simulink model "drone_pitch_test"  (R2025b)
settings: Solver=VariableStepAuto  StartTime=0.0  StopTime=3  RelTol=1e-3
libraries: sim3dcameralib x4, uavsim3dlib x4, sim3dautolib x1, sim3dlib x1
settings Model: Creator=lab  LastModifiedBy=lab

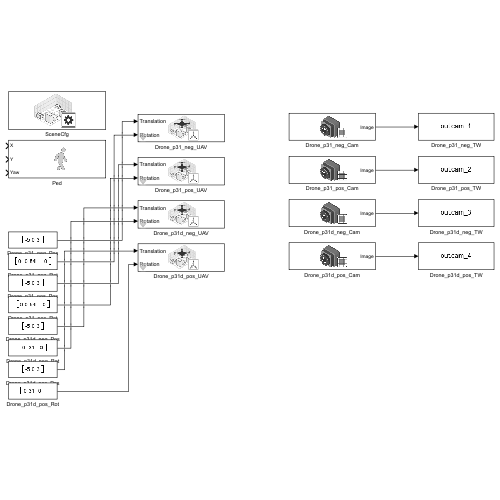
[thumbnail: Simulink's stored preview of the top-level diagram]
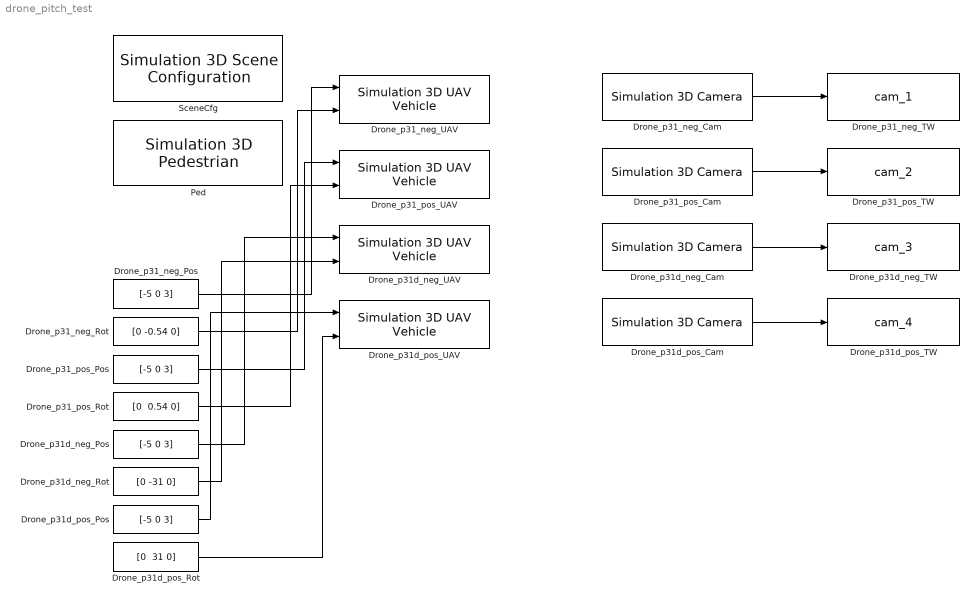
== system drone_pitch_test ==
  Drone_p31_neg_Cam : sim3dcameralib/Simulation 3D Camera  Priority=1  sensorTag=Sim3dSensor  sensorId=1  sensorName=Sim3dSensor  vehTagList={'Scene Origin', 'Drone_p31_neg'}  vehTag=Drone_p31_neg  CoordinateSystem=ISO8855  mountLoc=Origin  offsetFlag=on  tmountOffset=[0 0 0]  extTmount=off  rmountOffset=[0 0 0]  extRmount=off  FocalLength=[1109, 1109]  OpticalCenter=[640, 360]  ImageSize=[640 360]  RadialDistortion=[0, 0]  TangentialDistortion=[0, 0]  SensorSkew=0  VisualizeFieldOfView=off  FieldOfViewRange=61  DepthOutportEnabled=off  SemanticOutportEnabled=off  TransformOutportEnabled=off  SampleTime=0.5  mountPoint=[0 0 0]  mountOrientation=[0 0 0]  aMode=4  ID=1
      settings: LibrarySourceBlock=uavsim3dlib/Simulation 3D Camera
  Drone_p31_neg_Pos : Constant  Value=[-5 0 3]
  Drone_p31_neg_Rot : Constant  Value=[0 -0.54 0]
  Drone_p31_neg_TW : ToWorkspace  VariableName=cam_1  SaveFormat=Structure With Time  SampleTime=-1
  Drone_p31_neg_UAV : uavsim3dlib/Simulation 3D UAV Vehicle  Priority=-1  Mesh=Quadrotor  MeshPath=/MathWorksUAVContent/UAVs/HexaRotorUAV/HexaRotor.HexaRotor  Color=Red  ActorName=Drone_p31_neg  UseGlobalFrame=off  InitialTranslation=[-5 0 3]  InitialRotation=[0 -0.54 0]  InitialTranslationGlobal=[0 0 0]  InitialGeoOrigin=[0 0 0]  InitialRotationGlobal=[0 0 0]  SampleTime=-1  ActorType=SimulinkVehicle  ID=C  aMode=4  ActorTag=Drone_p31_neg
  Drone_p31_pos_Cam : sim3dcameralib/Simulation 3D Camera  Priority=1  sensorTag=Sim3dSensor  sensorId=2  sensorName=Sim3dSensor  vehTagList={'Scene Origin', 'Drone_p31_pos'}  vehTag=Drone_p31_pos  CoordinateSystem=ISO8855  mountLoc=Origin  offsetFlag=on  tmountOffset=[0 0 0]  extTmount=off  rmountOffset=[0 0 0]  extRmount=off  FocalLength=[1109, 1109]  OpticalCenter=[640, 360]  ImageSize=[640 360]  RadialDistortion=[0, 0]  TangentialDistortion=[0, 0]  SensorSkew=0  VisualizeFieldOfView=off  FieldOfViewRange=61  DepthOutportEnabled=off  SemanticOutportEnabled=off  TransformOutportEnabled=off  SampleTime=0.5  mountPoint=[0 0 0]  mountOrientation=[0 0 0]  aMode=4  ID=2
      settings: LibrarySourceBlock=uavsim3dlib/Simulation 3D Camera
  Drone_p31_pos_Pos : Constant  Value=[-5 0 3]
  Drone_p31_pos_Rot : Constant  Value="[0  0.54 0]"
  Drone_p31_pos_TW : ToWorkspace  VariableName=cam_2  SaveFormat=Structure With Time  SampleTime=-1
  Drone_p31_pos_UAV : uavsim3dlib/Simulation 3D UAV Vehicle  Priority=-1  Mesh=Quadrotor  MeshPath=/MathWorksUAVContent/UAVs/HexaRotorUAV/HexaRotor.HexaRotor  Color=Red  ActorName=Drone_p31_pos  UseGlobalFrame=off  InitialTranslation=[-5 0 3]  InitialRotation="[0  0.54 0]"  InitialTranslationGlobal=[0 0 0]  InitialGeoOrigin=[0 0 0]  InitialRotationGlobal=[0 0 0]  SampleTime=-1  ActorType=SimulinkVehicle  ID=C  aMode=4  ActorTag=Drone_p31_pos
  Drone_p31d_neg_Cam : sim3dcameralib/Simulation 3D Camera  Priority=1  sensorTag=Sim3dSensor  sensorId=3  sensorName=Sim3dSensor  vehTagList={'Scene Origin', 'Drone_p31d_neg'}  vehTag=Drone_p31d_neg  CoordinateSystem=ISO8855  mountLoc=Origin  offsetFlag=on  tmountOffset=[0 0 0]  extTmount=off  rmountOffset=[0 0 0]  extRmount=off  FocalLength=[1109, 1109]  OpticalCenter=[640, 360]  ImageSize=[640 360]  RadialDistortion=[0, 0]  TangentialDistortion=[0, 0]  SensorSkew=0  VisualizeFieldOfView=off  FieldOfViewRange=61  DepthOutportEnabled=off  SemanticOutportEnabled=off  TransformOutportEnabled=off  SampleTime=0.5  mountPoint=[0 0 0]  mountOrientation=[0 0 0]  aMode=4  ID=3
      settings: LibrarySourceBlock=uavsim3dlib/Simulation 3D Camera
  Drone_p31d_neg_Pos : Constant  Value=[-5 0 3]
  Drone_p31d_neg_Rot : Constant  Value=[0 -31 0]
  Drone_p31d_neg_TW : ToWorkspace  VariableName=cam_3  SaveFormat=Structure With Time  SampleTime=-1
  Drone_p31d_neg_UAV : uavsim3dlib/Simulation 3D UAV Vehicle  Priority=-1  Mesh=Quadrotor  MeshPath=/MathWorksUAVContent/UAVs/HexaRotorUAV/HexaRotor.HexaRotor  Color=Red  ActorName=Drone_p31d_neg  UseGlobalFrame=off  InitialTranslation=[-5 0 3]  InitialRotation=[0 -31 0]  InitialTranslationGlobal=[0 0 0]  InitialGeoOrigin=[0 0 0]  InitialRotationGlobal=[0 0 0]  SampleTime=-1  ActorType=SimulinkVehicle  ID=C  aMode=4  ActorTag=Drone_p31d_neg
  Drone_p31d_pos_Cam : sim3dcameralib/Simulation 3D Camera  Priority=1  sensorTag=Sim3dSensor  sensorId=4  sensorName=Sim3dSensor  vehTagList={'Scene Origin', 'Drone_p31d_pos'}  vehTag=Drone_p31d_pos  CoordinateSystem=ISO8855  mountLoc=Origin  offsetFlag=on  tmountOffset=[0 0 0]  extTmount=off  rmountOffset=[0 0 0]  extRmount=off  FocalLength=[1109, 1109]  OpticalCenter=[640, 360]  ImageSize=[640 360]  RadialDistortion=[0, 0]  TangentialDistortion=[0, 0]  SensorSkew=0  VisualizeFieldOfView=off  FieldOfViewRange=61  DepthOutportEnabled=off  SemanticOutportEnabled=off  TransformOutportEnabled=off  SampleTime=0.5  mountPoint=[0 0 0]  mountOrientation=[0 0 0]  aMode=4  ID=4
      settings: LibrarySourceBlock=uavsim3dlib/Simulation 3D Camera
  Drone_p31d_pos_Pos : Constant  Value=[-5 0 3]
  Drone_p31d_pos_Rot : Constant  Value="[0  31 0]"
  Drone_p31d_pos_TW : ToWorkspace  VariableName=cam_4  SaveFormat=Structure With Time  SampleTime=-1
  Drone_p31d_pos_UAV : uavsim3dlib/Simulation 3D UAV Vehicle  Priority=-1  Mesh=Quadrotor  MeshPath=/MathWorksUAVContent/UAVs/HexaRotorUAV/HexaRotor.HexaRotor  Color=Red  ActorName=Drone_p31d_pos  UseGlobalFrame=off  InitialTranslation=[-5 0 3]  InitialRotation="[0  31 0]"  InitialTranslationGlobal=[0 0 0]  InitialGeoOrigin=[0 0 0]  InitialRotationGlobal=[0 0 0]  SampleTime=-1  ActorType=SimulinkVehicle  ID=C  aMode=4  ActorTag=Drone_p31d_pos
  Ped : sim3dautolib/Simulation 3D Pedestrian  Priority=-1  PedestrianType=Male 1  Scale=[1, 1, 1]  CoordinateSystem=ISO8855  InitialPos=[0 0 0]  InitialYaw=0  ActorName=SimulinkPedestrian1  SampleTime=-1  ActorType=SimulinkPedestrian  ActorTag=SimulinkPedestrian1  ID=1  aMode=3  CoordinateScheme=0  TransformOutportEnabled=off
      settings: LibrarySourceBlock=drivingsim3d/Simulation 3D Pedestrian
  SceneCfg : sim3dlib/Simulation 3D Scene Configuration  Priority=0  ProjectFormat=Default Scenes  SceneDesc=Empty Grass  ProjectName=C:\Program Files\MATLAB\R2025b\toolbox\shared\sim3d_projects\automotive_project_windows\UE\WindowsNoEditor\VehicleSimulation.exe  ScenePath=/Game/Maps/USCityBlock  EnableOpenDRIVE=off  vehTagList={'Custom';'Scene Origin'}  vehTag=Scene Origin  AttachedCameraRelativeTranslation=[0 0 0]  FreeCameraDefaultInitialTranslation=[-6, 0, 2]  AttachedCameraRelativeRotation=[0 0 0]  FreeCameraDefaultInitialRotation=[0, -15, 0]  ViewpointName=Custom  FreeCameraInitialTranslation=[0, 0, 0]  ViewpointTranslation=[0, 0, 0]  FreeCameraInitialRotation=[0, 0, 0]  ViewpointRotation=[0, 0, 0]  OpVisEn=off  Ts=1/60  EnableWindow=on  EnableRemoteAccess=off  EnableWeather=off  SunAzimuth=90  SunAltitude=40.0  EnableGeospatialSun=off  Latitude=0  Longitude=0  Date=2023-01-01  Time=10:30:00  GeoTimeZone=-5.0  SunDaylightSaving=off  wind=1  clouds=10  EnableVolumetricClouds=off  CloudCoverage=0  CloudAltitude=6  fog=0  rain=0  RaindropsEffect=off  SnowDensity=0  EnableGeospatial=off  TilesetSource=Earth terrain  UseTrueOrigin=off  OriginHeight=200  OriginLatitude=40.744652  OriginLongitude=-73.988864  MapStyle=Aerial  AdditionalAssetIDs=[]  UseAdvancedSunSky=off  SolarTime=11  TimeZone=-5  Day=21  Month=9  Year=2022  UseDaylightSavingTime=on  DSTStartDay=10  DSTStartMonth=3  DSTEndDay=3  DSTEndMonth=11  DSTSwitchHour=2  sensorTag=MainCamera1  sensorId=1  sensorName=MainCamera1  mountLoc=Origin  offsetFlag=off  tmountOffset=[0, 0, 0]  rmountOffset=[0, 0, 0]  HorizontalResolution=1280  VerticalResolution=720  HorizontalFOV=60  mountPoint=[0 0 0]  mountOrientation=[0 0 0]  aMode=4  ID=1  GeoTrigger=Inactive  ViewNameList={'Custom'}  ViewTranslationList={'[0 0 0]'}  ViewRotationList={'[0 0 0]'}
      settings: LibrarySourceBlock=uavsim3dlib/Simulation 3D Scene Configuration
  wires:
  Drone_p31_neg_Pos/1 -> Drone_p31_neg_UAV/1
  Drone_p31_neg_Rot/1 -> Drone_p31_neg_UAV/2
  Drone_p31_pos_Pos/1 -> Drone_p31_pos_UAV/1
  Drone_p31_pos_Rot/1 -> Drone_p31_pos_UAV/2
  Drone_p31d_neg_Pos/1 -> Drone_p31d_neg_UAV/1
  Drone_p31d_neg_Rot/1 -> Drone_p31d_neg_UAV/2
  Drone_p31d_pos_Pos/1 -> Drone_p31d_pos_UAV/1
  Drone_p31d_pos_Rot/1 -> Drone_p31d_pos_UAV/2
  Drone_p31_neg_Cam/1 -> Drone_p31_neg_TW/1
  Drone_p31_pos_Cam/1 -> Drone_p31_pos_TW/1
  Drone_p31d_neg_Cam/1 -> Drone_p31d_neg_TW/1
  Drone_p31d_pos_Cam/1 -> Drone_p31d_pos_TW/1
